simulink model "untitled"  (Simulink 7.9)
settings: Solver=ode45  StartTime=0.0  StopTime=50  MaxStep=0.04  RelTol=1e-3
settings Model: Creator=aziemba  LastModifiedBy=aziemba

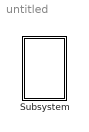
== system untitled ==
  Subsystem : Subsystem  mask{g=9.81, m1=1, m2=3, m=1, R=0.01, r0=1, fi0=90}

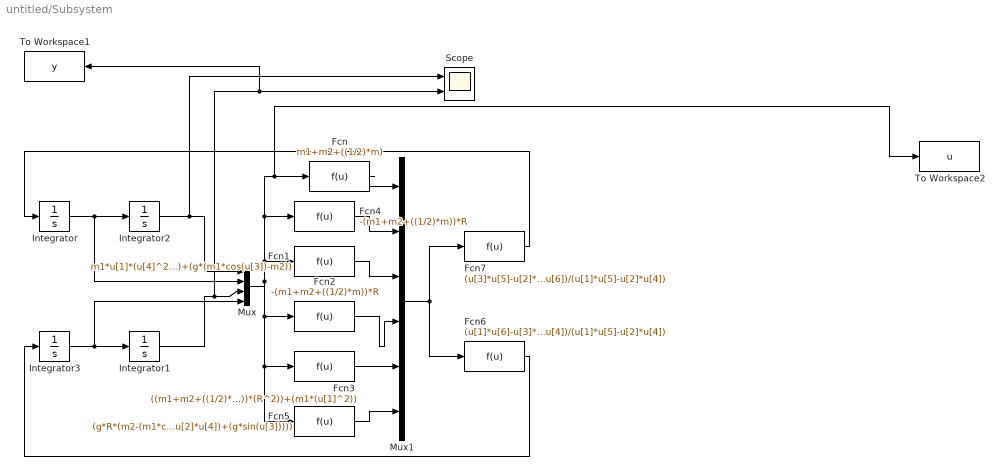
== system untitled/Subsystem ==
  Fcn : Fcn  Expr=m1+m2+((1/2)*m)
  Fcn1 : Fcn  Expr=m1*u[1]*(u[4]^2)+(g*(m1*cos(u[3])-m2))
  Fcn2 : Fcn  Expr=-(m1+m2+((1/2)*m))*R
  Fcn3 : Fcn  Expr=((m1+m2+((1/2)*m))*(R^2))+(m1*(u[1]^2))
  Fcn4 : Fcn  Expr=-(m1+m2+((1/2)*m))*R
  Fcn5 : Fcn  Expr=(g*R*(m2-(m1*cos(u[3]))))-(m1*u[1]*((2*u[2]*u[4])+(g*sin(u[3]))))
  Fcn6 : Fcn  Expr=(u[1]*u[6]-u[3]*u[4])/(u[1]*u[5]-u[2]*u[4])
  Fcn7 : Fcn  Expr=(u[3]*u[5]-u[2]*u[6])/(u[1]*u[5]-u[2]*u[4])
  Integrator : Integrator
  Integrator1 : Integrator  InitialCondition=(fi0*pi)/180
  Integrator2 : Integrator  InitialCondition=r0
  Integrator3 : Integrator
  Mux : Mux
  Mux1 : Mux  Inputs=6
  Scope : Scope  NumInputPorts=2
      settings: YMin=-5~-5  YMax=5~5
  To Workspace1 : ToWorkspace  VariableName=y  SampleTime=-1
  To Workspace2 : ToWorkspace  VariableName=u  SampleTime=-1
  wires:
  Integrator3/1 -> Integrator1/1, Mux/4
  Integrator/1 -> Integrator2/1, Mux/2
  Integrator1/1 -> Mux/3, Scope/2, To Workspace1/1
  Integrator2/1 -> Mux/1, Scope/1
  Mux/1 -> Fcn4/1, Fcn/1, To Workspace2/1, Fcn1/1, Fcn5/1, Fcn3/1, Fcn2/1
  Fcn/1 -> Mux1/1
  Fcn4/1 -> Mux1/2
  Fcn1/1 -> Mux1/3
  Fcn5/1 -> Mux1/6
  Mux1/1 -> Fcn7/1, Fcn6/1
  Fcn7/1 -> Integrator/1
  Fcn6/1 -> Integrator3/1
  Fcn2/1 -> Mux1/4
  Fcn3/1 -> Mux1/5
